simulink model "sensorFusion__impl_1"  (R2017b)
settings: Solver=FixedStepDiscrete  StartTime=0.0  StopTime=10.0  FixedStep=1  RelTol=1e-3
model mask{LongRangeRadarUpperLimit=LongRangeRadarUpperLimit, ShortRangeRadarUpperLimit=ShortRangeRadarUpperLimit}
PreLoadFcn:
  | sl_refresh_customizations
  | enum_Simulink
  | simulinkExportUnitCs
  | ACC_Parameters
  | ACCData
InitFcn:
  | checkUnitMismatch
model workspace (MAT data in the model file):
  ESD_URL = 'http://127.0.0.1:63320/node?ref=r%3Af6839c77-5b9d-441b-9a46-8668f7352d69%28A_ACC._50_ImplementationDefinitionHeterogeneous%29%2F2271559521715991060'
  LongRangeRadarUpperLimit = Simulink.Parameter
  LongRangeRadarUpperLimit.Value = 0
  LongRangeRadarUpperLimit.DataType = 'double'
  LongRangeRadarUpperLimit.DocUnits = 'm'
  LongRangeRadarUpperLimit.Dimensions = [1 1]
  ModelMaskData(1).paramName = 'LongRangeRadarUpperLimit'
  ModelMaskData(1).paramType = 'double /m/'
  ModelMaskData(1).promptString = 'LongRangeRadarUpperLimit(datatype: double, unit:m)'
  ModelMaskData(2).paramName = 'ShortRangeRadarUpperLimit'
  ModelMaskData(2).paramType = 'double /cm/'
  ModelMaskData(2).promptString = 'ShortRangeRadarUpperLimit(datatype: double, unit:cm)'
  ShortRangeRadarUpperLimit = Simulink.Parameter
  ShortRangeRadarUpperLimit.Value = 0
  ShortRangeRadarUpperLimit.DataType = 'double'
  ShortRangeRadarUpperLimit.DocUnits = 'cm'
  ShortRangeRadarUpperLimit.Dimensions = [1 1]
settings Model: ParameterArgumentNames=LongRangeRadarUpperLimit,ShortRangeRadarUpperLimit  Creator=eh6qym  LastModifiedBy=eh6qym
settings OptimizationCC: DefaultParameterBehavior=Inlined  PassReuseOutputArgsAs=Individual arguments  ZeroExternalMemoryAtStartup=off
settings DebuggingCC: SignalRangeChecking=error  InheritedTsInSrcMsg=none  ParameterTunabilityLossMsg=error
settings SFSimCC: MATLABDynamicMemAlloc=off
settings RTWCC: SystemTargetFile=esd_ert.tlc  GenCodeOnly=on  TemplateMakefile=ert_default_tmf  Description=CSD  GenerateReport=on  IncludeHyperlinkInReport=on  LaunchReport=on  GenerateTraceInfo=on  GenerateTraceReport=on  GenerateTraceReportSl=on  GenerateTraceReportSf=on  GenerateTraceReportEml=on
settings CodeAppCC: ForceParamTrailComments=on  IgnoreCustomStorageClasses=off  OperatorAnnotations=on  SimulinkDataObjDesc=on  SFDataObjDesc=on  InsertBlockDesc=on
settings STFCustomTargetCC: TargetLangStandard=C99 (ISO)  MultiwordLength=256  GenerateSampleERTMain=on  IncludeMdlTerminateFcn=off  CombineOutputUpdateFcns=on  CombineSignalStateStructs=on  SuppressErrorStatus=on  ERTCustomFileBanners=on  MultiInstanceERTCode=on  CodeInterfacePackaging=Reusable function  SupportContinuousTime=off  SupportNonInlinedSFcns=off  RemoveDisableFunc=on  RemoveResetFunc=on  MATLABClassNameForMDSCustomization=Simulink.SoftwareTarget.ERTCustomization  GRTInterface=off  SystemTargetFile=esd_ert.tlc
settings ERTTargetCC: TargetLangStandard=C99 (ISO)  GenerateSampleERTMain=on  ParMdlRefBuildCompliant=off  CompOptLevelCompliant=off  ConcurrentExecutionCompliant=off  IncludeMdlTerminateFcn=off  CombineSignalStateStructs=on  SuppressErrorStatus=on  MultiInstanceERTCode=on  CodeInterfacePackaging=Reusable function  RemoveDisableFunc=on  ModelStepFunctionPrototypeControlCompliant=off  CPPClassGenCompliant=off  UseToolchainInfoCompliant=off  InlinedParameterPlacement=NonHierarchical  ERTCustomFileTemplate=example_file_process.tlc

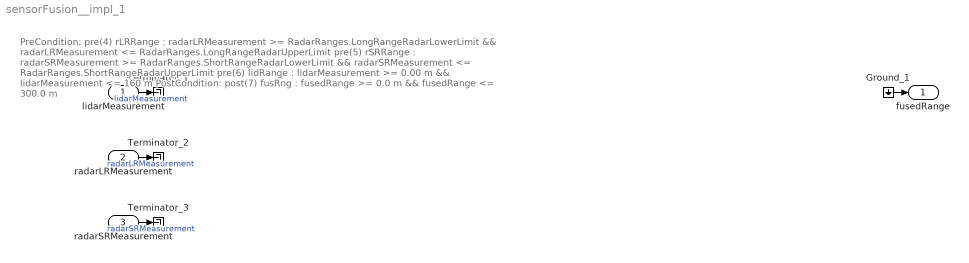
== system sensorFusion__impl_1 ==
  note: PreCondition:
      | pre(4) rLRRange :   radarLRMeasurement >= RadarRanges.LongRangeRadarLowerLimit && radarLRMeasurement <= RadarRanges.LongRangeRadarUpperLimit
      | pre(5) rSRRange :   radarSRMeasurement >= RadarRanges.ShortRangeRadarLowerLimit && radarSRMeasurement <= RadarRanges.ShortRangeRadarUpperLimit
      | pre(6) lidRange :   lidarMeasurement >= 0.00 m && lidarMeasurement <= 160 m
      | PostCondition:
      | post(7) fusRng :   fusedRange >= 0.0 m && fusedRange <= 300.0 m
  lidarMeasurement : Inport  OutDataTypeStr=double  Unit=m
      settings: AttributesFormatString=(m)
  radarLRMeasurement : Inport  Port=2  OutDataTypeStr=double  Unit=m
      settings: AttributesFormatString=(m)
  radarSRMeasurement : Inport  Port=3  OutDataTypeStr=double  Unit=cm
      settings: AttributesFormatString=(cm)
  Ground_1 : Ground
  Terminator_1 : Terminator
  Terminator_2 : Terminator
  Terminator_3 : Terminator
  fusedRange : Outport  OutDataTypeStr=double  Unit=m
      settings: AttributesFormatString=(m)
  wires:
  lidarMeasurement/1 -> Terminator_1/1  "lidarMeasurement"
  radarLRMeasurement/1 -> Terminator_2/1  "radarLRMeasurement"
  radarSRMeasurement/1 -> Terminator_3/1  "radarSRMeasurement"
  Ground_1/1 -> fusedRange/1
